simulink model "Trimmodel"  (R2023b)
settings: Solver=ode4  StartTime=0.0  StopTime=100  FixedStep=1e-3  RelTol=1e-3
undefined symbols (not defined in the file or in its folder): Aeroparams, Aircraftparams, Atmosphereparams, Inertiaconstants, Initialconds, Propparams
libraries: simulink_extras x25
(part 3 of 3)

== system Trimmodel/NonlinearF16Model/Simframe/Rigidbodydynamics/Kinematicequations/Eulerlimitations/merge ==
  In1 : Inport
  In2 : Inport  Port=2
  In3 : Inport  Port=3
  In4 : Inport  Port=4
  In5 : Inport  Port=5
  In6 : Inport  Port=6
  In7 : Inport  Port=7
  In8 : Inport  Port=8
  In9 : Inport  Port=9
  In10 : Inport  Port=10
  In11 : Inport  Port=11
  In12 : Inport  Port=12
  In13 : Inport  Port=13
  In14 : Inport  Port=14
  In15 : Inport  Port=15
  Merge : Merge  Inputs=5
  Merge1 : Merge  Inputs=5
  Merge2 : Merge  Inputs=5
  Out1 : Outport
  Outport : Outport  Port=2
  Out3 : Outport  Port=3
  wires:
  Merge/1 -> Outport/1  "theta"
  Merge1/1 -> Out1/1  "phi"
  Merge2/1 -> Out3/1  "psi"
  In1/1 -> Merge1/1
  In4/1 -> Merge1/2
  In7/1 -> Merge1/3
  In10/1 -> Merge1/4
  In13/1 -> Merge1/5
  In2/1 -> Merge/1
  In5/1 -> Merge/2
  In8/1 -> Merge/3
  In11/1 -> Merge/4
  In14/1 -> Merge/5
  In3/1 -> Merge2/1
  In6/1 -> Merge2/2
  In9/1 -> Merge2/3
  In12/1 -> Merge2/4
  In15/1 -> Merge2/5

== system Trimmodel/NonlinearF16Model/Simframe/Rigidbodydynamics/Kinematicequations/kinematicequationseulerdot/Avoidsingularity ==
  note: Input assignment
  note: To avoid singularity limit theta to +89.99° / -89.99° | +90.01° / -90.01°
  theta : Inport
  thetadot : Inport  Port=2
  Constant : Constant  Value=89.99
  Constant1 : Constant  Value=-89.99
  Constant2 : Constant  Value=90.01
  Constant3 : Constant  Value=-90.01
  Constant4 : Constant  Value=90
  Constant5 : Constant  Value=-90
  Degrees to Radians{,1..5} (6 alike) : simulink_extras/Transformations/Degrees to Radians
  If : If  NumInputs=7  IfExpression=u1 > u2 & u1 < u6  ElseIfExpressions=u1 > u6 & u1 < u4 , u1 < u3 & u1 > u7 , u1 < u7 & u1 > u5 , u1 == u6 , u1 == u7
  If Action Subsystem : Subsystem
  If Action Subsystem1 : Subsystem
  If Action Subsystem2 : Subsystem
  If Action Subsystem3 : Subsystem
  If Action Subsystem4 : Subsystem
  If Action Subsystem5 : Subsystem
  If Action Subsystem6 : Subsystem
  Merge : Merge  Inputs=7
  Outport : Outport
  wires:
  If Action Subsystem2/1(Out1) -> Merge/7
  If Action Subsystem6/1(theta) -> Merge/6
  If Action Subsystem5/1(theta) -> Merge/5
  [thetadot] -> If Action Subsystem5/1(thetadot)
  [thetadot] -> If Action Subsystem6/1(thetadot)
  thetadot/1 -> [thetadot]
  If/6 -> If Action Subsystem6/Action
  If/5 -> If Action Subsystem5/Action
  If/7 -> If Action Subsystem2/Action
  If/4 -> If Action Subsystem1/Action
  If/3 -> If Action Subsystem4/Action
  If/2 -> If Action Subsystem3/Action
  If/1 -> If Action Subsystem/Action
  If Action Subsystem1/1(theta) -> Merge/4
  If Action Subsystem3/1(theta) -> Merge/2
  If Action Subsystem/1(theta) -> Merge/1
  If Action Subsystem4/1(theta) -> Merge/3
  Degrees to Radians5/1 -> If/7
  Constant5/1 -> Degrees to Radians5/1
  Degrees to Radians4/1 -> If/6
  Constant4/1 -> Degrees to Radians4/1
  Degrees to Radians3/1 -> If/5
  Constant3/1 -> Degrees to Radians3/1
  Constant2/1 -> Degrees to Radians2/1
  Degrees to Radians2/1 -> If/4
  theta/1 -> If Action Subsystem2/1(theta), If/1
  Merge/1 -> Outport/1  "theta"
  Constant/1 -> Degrees to Radians/1
  Degrees to Radians/1 -> If/2
  Degrees to Radians1/1 -> If/3
  Constant1/1 -> Degrees to Radians1/1

== system Trimmodel/NonlinearF16Model/Simframe/Rigidbodydynamics/Kinematicequations/kinematicequationseulerdot/kinematicequationstfmatrix ==
  note: Input assignment
  <phi> : Inport
  <theta> : Inport  Port=2
  Cos : Trigonometry  Operator=tan
  Cos3 : Trigonometry  Operator=cos
  Cos4 : Trigonometry  Operator=cos
  Cos5 : Trigonometry
  Firstrow : Subsystem
  Matrix Concatenate : Concatenate  NumInputs=3  Mode=Multidimensional array
  secondrow : Subsystem
  thirdrow : Subsystem
  transformationmatrix : Outport
  wires:
  [sinphi] -> thirdrow/1(sinphi)
  [costheta] -> thirdrow/3(costheta)
  [cosphi] -> thirdrow/2(cosphi)
  secondrow/1(secondrow) -> Matrix Concatenate/2
  [cosphi] -> secondrow/2(cosphi)
  [sinphi] -> secondrow/1(sinphi)
  [sinphi] -> Firstrow/2(sinphi)
  [cosphi] -> Firstrow/3(cosphi)
  [tantheta] -> Firstrow/1(tantheta)
  Matrix Concatenate/1 -> transformationmatrix/1
  thirdrow/1(thirdrow) -> Matrix Concatenate/3
  Firstrow/1(firstrow) -> Matrix Concatenate/1
  Cos3/1 -> [costheta]
  Cos/1 -> [tantheta]
  Cos5/1 -> [sinphi]
  Cos4/1 -> [cosphi]
  <phi>/1 -> Cos4/1, Cos5/1
  <theta>/1 -> Cos/1, Cos3/1

== system Trimmodel/NonlinearF16Model/Simframe/Rigidbodydynamics/Navigationequations/navigationequationstfmatrix/firstrow ==
  note: Input assignment
  cosphi : Inport
  sinphi : Inport  Port=2
  costheta : Inport  Port=3
  sintheta : Inport  Port=4
  cospsi : Inport  Port=5
  sinpsi : Inport  Port=6
  Add1 : Sum  Inputs=+-
  Add2 : Sum
  Divide1 : Product  Inputs=**
  Divide2 : Product  Inputs=***
  Divide3 : Product  Inputs=***
  Divide4 : Product  Inputs=**
  Divide5 : Product  Inputs=**
  Vector Concatenate : Concatenate  NumInputs=3  Mode=Multidimensional array  ConcatenateDimension=2
  firstrow : Outport
  wires:
  Vector Concatenate/1 -> firstrow/1
  Divide1/1 -> Vector Concatenate/1
  Add1/1 -> Vector Concatenate/2
  sinpsi/1 -> [sinpsi]
  [sinphi] -> Divide3/1
  [sintheta] -> Divide3/2
  [cospsi] -> Divide3/3
  Divide3/1 -> Add1/1
  [cosphi] -> Divide4/1
  [sinpsi] -> Divide4/2
  Divide4/1 -> Add1/2
  [cospsi] -> Divide1/2
  [costheta] -> Divide1/1
  cospsi/1 -> [cospsi]
  cosphi/1 -> [cosphi]
  sinphi/1 -> [sinphi]
  sintheta/1 -> [sintheta]
  costheta/1 -> [costheta]
  Divide5/1 -> Add2/2
  [sinpsi] -> Divide5/2
  [sinphi] -> Divide5/1
  Divide2/1 -> Add2/1
  [cospsi] -> Divide2/3
  [sintheta] -> Divide2/2
  [cosphi] -> Divide2/1
  Add2/1 -> Vector Concatenate/3

== system Trimmodel/NonlinearF16Model/Simframe/Rigidbodydynamics/Navigationequations/navigationequationstfmatrix/secondrow ==
  note: Input assignment
  cosphi : Inport
  sinphi : Inport  Port=2
  costheta : Inport  Port=3
  sintheta : Inport  Port=4
  cospsi : Inport  Port=5
  sinpsi : Inport  Port=6
  Add1 : Sum
  Add2 : Sum  Inputs=+-
  Divide1 : Product  Inputs=**
  Divide2 : Product  Inputs=***
  Divide3 : Product  Inputs=***
  Divide4 : Product  Inputs=**
  Divide5 : Product  Inputs=**
  Vector Concatenate : Concatenate  NumInputs=3  Mode=Multidimensional array  ConcatenateDimension=2
  secondrow : Outport
  wires:
  Add2/1 -> Vector Concatenate/3
  [cosphi] -> Divide2/1
  [sintheta] -> Divide2/2
  [sinpsi] -> Divide2/3
  Divide2/1 -> Add2/1
  [sinphi] -> Divide5/1
  [cospsi] -> Divide5/2
  Divide5/1 -> Add2/2
  costheta/1 -> [costheta]
  sintheta/1 -> [sintheta]
  sinphi/1 -> [sinphi]
  cosphi/1 -> [cosphi]
  cospsi/1 -> [cospsi]
  [costheta] -> Divide1/1
  [sinpsi] -> Divide1/2
  Divide4/1 -> Add1/2
  [cospsi] -> Divide4/2
  [cosphi] -> Divide4/1
  Divide3/1 -> Add1/1
  [sinpsi] -> Divide3/3
  [sintheta] -> Divide3/2
  [sinphi] -> Divide3/1
  sinpsi/1 -> [sinpsi]
  Add1/1 -> Vector Concatenate/2
  Divide1/1 -> Vector Concatenate/1
  Vector Concatenate/1 -> secondrow/1

== system Trimmodel/NonlinearF16Model/Simframe/Rigidbodydynamics/Navigationequations/navigationequationstfmatrix/thirdrow ==
  note: Input assignment
  cosphi : Inport
  sinphi : Inport  Port=2
  costheta : Inport  Port=3
  sintheta : Inport  Port=4
  Divide3 : Product  Inputs=**
  Divide5 : Product  Inputs=**
  Gain : Gain  Gain=-1
  Vector Concatenate : Concatenate  NumInputs=3  Mode=Multidimensional array  ConcatenateDimension=2
  thirdrow : Outport
  wires:
  Vector Concatenate/1 -> thirdrow/1
  Gain/1 -> Vector Concatenate/1
  [sinphi] -> Divide3/1
  [costheta] -> Divide3/2
  [sintheta] -> Gain/1
  cosphi/1 -> [cosphi]
  sinphi/1 -> [sinphi]
  sintheta/1 -> [sintheta]
  costheta/1 -> [costheta]
  [costheta] -> Divide5/2
  [cosphi] -> Divide5/1
  Divide3/1 -> Vector Concatenate/2
  Divide5/1 -> Vector Concatenate/3

== system Trimmodel/NonlinearF16Model/Airframe/Propulsion/Padot/propmodeltauPc/If Action Subsystem1/If Action Subsystem ==
  Action Port : ActionPort  ActionPortLabel=if(u1 <= 25)
  Constant : Constant
  tau : Outport
  wires:
  Constant/1 -> tau/1

== system Trimmodel/NonlinearF16Model/Airframe/Propulsion/Padot/propmodeltauPc/If Action Subsystem1/If Action Subsystem1 ==
  Action Port : ActionPort  ActionPortLabel=elseif(u1 >= 50)
  Constant : Constant  Value=0.1
  tau : Outport
  wires:
  Constant/1 -> tau/1

== system Trimmodel/NonlinearF16Model/Airframe/Propulsion/Padot/propmodeltauPc/If Action Subsystem1/If Action Subsystem2 ==
  dP : Inport
  Action Port : ActionPort  ActionPortLabel=else
  Add : Sum  Inputs=+-
  Constant : Constant  Value=1.9
  Gain : Gain  Gain=0.036
  tau : Outport
  wires:
  Add/1 -> tau/1
  Gain/1 -> Add/2
  dP/1 -> Gain/1
  Constant/1 -> Add/1

== system Trimmodel/NonlinearF16Model/Airframe/Propulsion/Padot/propmodeltauPc/If Action Subsystem2/If Action Subsystem ==
  Action Port : ActionPort  ActionPortLabel=if(u1 <= 25)
  Constant : Constant
  tau : Outport
  wires:
  Constant/1 -> tau/1

== system Trimmodel/NonlinearF16Model/Airframe/Propulsion/Padot/propmodeltauPc/If Action Subsystem2/If Action Subsystem1 ==
  Action Port : ActionPort  ActionPortLabel=elseif(u1 >= 50)
  Constant : Constant  Value=0.1
  tau : Outport
  wires:
  Constant/1 -> tau/1

== system Trimmodel/NonlinearF16Model/Airframe/Propulsion/Padot/propmodeltauPc/If Action Subsystem2/If Action Subsystem2 ==
  dP : Inport
  Action Port : ActionPort  ActionPortLabel=else
  Add : Sum  Inputs=+-
  Constant : Constant  Value=1.9
  Gain : Gain  Gain=0.036
  tau : Outport
  wires:
  Add/1 -> tau/1
  Gain/1 -> Add/2
  dP/1 -> Gain/1
  Constant/1 -> Add/1

== system Trimmodel/NonlinearF16Model/Simframe/Rigidbodydynamics/Kinematicequations/Eulerlimitations/Phi/If Action Subsystem ==
  phi : Inport
  Action Port : ActionPort  ActionPortLabel=if(u1 >= u2)
  Add : Sum  Inputs=+-
  Constant : Constant  Value=2*pi
  Out1 : Outport
  wires:
  phi/1 -> Add/1
  Constant/1 -> Add/2
  Add/1 -> Out1/1  "phi"

== system Trimmodel/NonlinearF16Model/Simframe/Rigidbodydynamics/Kinematicequations/Eulerlimitations/Phi/If Action Subsystem1 ==
  phi : Inport
  Action Port : ActionPort  ActionPortLabel=elseif(u1 < u3)
  Add : Sum
  Constant : Constant  Value=2*pi
  Out1 : Outport
  wires:
  Constant/1 -> Add/2
  Add/1 -> Out1/1  "phi"
  phi/1 -> Add/1

== system Trimmodel/NonlinearF16Model/Simframe/Rigidbodydynamics/Kinematicequations/Eulerlimitations/Phi/If Action Subsystem2 ==
  phi : Inport
  Action Port : ActionPort  ActionPortLabel=else
  Out1 : Outport
  wires:
  phi/1 -> Out1/1  "phi"

== system Trimmodel/NonlinearF16Model/Simframe/Rigidbodydynamics/Kinematicequations/Eulerlimitations/Psi/If Action Subsystem ==
  psi : Inport
  Action Port : ActionPort  ActionPortLabel=if(u1 >= u2)
  Add : Sum  Inputs=+-
  Constant : Constant  Value=2*pi
  Out1 : Outport
  wires:
  Add/1 -> Out1/1  "psi"
  Constant/1 -> Add/2
  psi/1 -> Add/1

== system Trimmodel/NonlinearF16Model/Simframe/Rigidbodydynamics/Kinematicequations/Eulerlimitations/Psi/If Action Subsystem1 ==
  psi : Inport
  Action Port : ActionPort  ActionPortLabel=elseif(u1 < u3)
  Add : Sum
  Constant : Constant  Value=2*pi
  Out1 : Outport
  wires:
  psi/1 -> Add/1
  Add/1 -> Out1/1  "psi"
  Constant/1 -> Add/2

== system Trimmodel/NonlinearF16Model/Simframe/Rigidbodydynamics/Kinematicequations/Eulerlimitations/Psi/If Action Subsystem2 ==
  psi : Inport
  Action Port : ActionPort  ActionPortLabel=else
  Out1 : Outport
  wires:
  psi/1 -> Out1/1  "psi"

== system Trimmodel/NonlinearF16Model/Simframe/Rigidbodydynamics/Kinematicequations/kinematicequationseulerdot/Avoidsingularity/If Action Subsystem ==
  Action Port : ActionPort  ActionPortLabel=if(u1 > u2 & u1 < u6)
  Constant : Constant  Value=89.99
  Degrees to Radians : simulink_extras/Transformations/Degrees to Radians
  theta : Outport
  wires:
  Constant/1 -> Degrees to Radians/1
  Degrees to Radians/1 -> theta/1

== system Trimmodel/NonlinearF16Model/Simframe/Rigidbodydynamics/Kinematicequations/kinematicequationseulerdot/Avoidsingularity/If Action Subsystem1 ==
  Action Port : ActionPort  ActionPortLabel=elseif( u1 < u7 & u1 > u5 )
  Constant : Constant  Value=-90.01
  Degrees to Radians : simulink_extras/Transformations/Degrees to Radians
  theta : Outport
  wires:
  Constant/1 -> Degrees to Radians/1
  Degrees to Radians/1 -> theta/1

== system Trimmodel/NonlinearF16Model/Simframe/Rigidbodydynamics/Kinematicequations/kinematicequationseulerdot/Avoidsingularity/If Action Subsystem2 ==
  theta : Inport
  Action Port : ActionPort  ActionPortLabel=else
  Out1 : Outport
  wires:
  theta/1 -> Out1/1  "theta"

== system Trimmodel/NonlinearF16Model/Simframe/Rigidbodydynamics/Kinematicequations/kinematicequationseulerdot/Avoidsingularity/If Action Subsystem3 ==
  Action Port : ActionPort  ActionPortLabel=elseif(u1 > u6 & u1 < u4 )
  Constant : Constant  Value=90.01
  Degrees to Radians : simulink_extras/Transformations/Degrees to Radians
  theta : Outport
  wires:
  Degrees to Radians/1 -> theta/1
  Constant/1 -> Degrees to Radians/1

== system Trimmodel/NonlinearF16Model/Simframe/Rigidbodydynamics/Kinematicequations/kinematicequationseulerdot/Avoidsingularity/If Action Subsystem4 ==
  Action Port : ActionPort  ActionPortLabel=elseif( u1 < u3 & u1 > u7 )
  Constant : Constant  Value=-89.99
  Degrees to Radians : simulink_extras/Transformations/Degrees to Radians
  theta : Outport
  wires:
  Constant/1 -> Degrees to Radians/1
  Degrees to Radians/1 -> theta/1

== system Trimmodel/NonlinearF16Model/Simframe/Rigidbodydynamics/Kinematicequations/kinematicequationseulerdot/Avoidsingularity/If Action Subsystem5 ==
  thetadot : Inport
  Action Port : ActionPort  ActionPortLabel=elseif( u1 == u6 )
  Constant : Constant  Value=89.99
  Constant1 : Constant  Value=90.01
  Degrees to Radians : simulink_extras/Transformations/Degrees to Radians
  Switch : Switch  Criteria=u2 > Threshold  SaturateOnIntegerOverflow=off  InputSameDT=off
  theta : Outport
  wires:
  Constant1/1 -> Switch/3
  Constant/1 -> Switch/1
  Switch/1 -> Degrees to Radians/1
  thetadot/1 -> Switch/2
  Degrees to Radians/1 -> theta/1

== system Trimmodel/NonlinearF16Model/Simframe/Rigidbodydynamics/Kinematicequations/kinematicequationseulerdot/Avoidsingularity/If Action Subsystem6 ==
  thetadot : Inport
  Action Port : ActionPort  ActionPortLabel=elseif( u1 == u7)
  Constant : Constant  Value=-90.01
  Constant1 : Constant  Value=-89.99
  Degrees to Radians : simulink_extras/Transformations/Degrees to Radians
  Switch : Switch  Criteria=u2 > Threshold  SaturateOnIntegerOverflow=off  InputSameDT=off
  theta : Outport
  wires:
  Degrees to Radians/1 -> theta/1
  Constant1/1 -> Switch/3
  thetadot/1 -> Switch/2
  Switch/1 -> Degrees to Radians/1
  Constant/1 -> Switch/1

== system Trimmodel/NonlinearF16Model/Simframe/Rigidbodydynamics/Kinematicequations/kinematicequationseulerdot/kinematicequationstfmatrix/Firstrow ==
  note: Input assignment
  tantheta : Inport
  sinphi : Inport  Port=2
  cosphi : Inport  Port=3
  Constant : Constant
  Divide1 : Product  Inputs=**
  Divide2 : Product  Inputs=**
  Vector Concatenate : Concatenate  NumInputs=3  Mode=Multidimensional array  ConcatenateDimension=2
  firstrow : Outport
  wires:
  [tantheta] -> Divide1/2
  Vector Concatenate/1 -> firstrow/1
  Divide1/1 -> Vector Concatenate/3
  Divide2/1 -> Vector Concatenate/2
  Constant/1 -> Vector Concatenate/1
  [cosphi] -> Divide1/1
  [tantheta] -> Divide2/2
  [sinphi] -> Divide2/1
  cosphi/1 -> [cosphi]
  sinphi/1 -> [sinphi]
  tantheta/1 -> [tantheta]

== system Trimmodel/NonlinearF16Model/Simframe/Rigidbodydynamics/Kinematicequations/kinematicequationseulerdot/kinematicequationstfmatrix/secondrow ==
  note: Input assignment
  sinphi : Inport
  cosphi : Inport  Port=2
  Constant : Constant  Value=0
  Gain : Gain  Gain=-1
  Vector Concatenate : Concatenate  NumInputs=3  Mode=Multidimensional array  ConcatenateDimension=2
  secondrow : Outport
  wires:
  sinphi/1 -> [sinphi]
  cosphi/1 -> [cosphi]
  [sinphi] -> Gain/1
  Constant/1 -> Vector Concatenate/1
  [cosphi] -> Vector Concatenate/2
  Gain/1 -> Vector Concatenate/3
  Vector Concatenate/1 -> secondrow/1

== system Trimmodel/NonlinearF16Model/Simframe/Rigidbodydynamics/Kinematicequations/kinematicequationseulerdot/kinematicequationstfmatrix/thirdrow ==
  note: Input assignment
  sinphi : Inport
  cosphi : Inport  Port=2
  costheta : Inport  Port=3
  Constant : Constant  Value=0
  Divide1 : Product  Inputs=*/
  Divide2 : Product  Inputs=*/
  Vector Concatenate : Concatenate  NumInputs=3  Mode=Multidimensional array  ConcatenateDimension=2
  thirdrow : Outport
  wires:
  [costheta] -> Divide1/2
  [costheta] -> Divide2/2
  sinphi/1 -> [sinphi]
  cosphi/1 -> [cosphi]
  costheta/1 -> [costheta]
  [sinphi] -> Divide2/1
  [cosphi] -> Divide1/1
  Constant/1 -> Vector Concatenate/1
  Divide2/1 -> Vector Concatenate/2
  Divide1/1 -> Vector Concatenate/3
  Vector Concatenate/1 -> thirdrow/1
